simulink model "example12_3"  (R2023b)
settings: Solver=FixedStepAuto  StartTime=0.0  StopTime=1000  FixedStep=0.01  RelTol=1e-3
InitFcn:
  | example12_3_param;
values from neighbouring files (symbols this model uses):
  A = [1 1 ; 0 1]    [example12_3_param.m]
  B = [0 ; 1]    [example12_3_param.m]
  Bw = [1; 1]    [example12_3_param.m]
  C = [1 0]    [example12_3_param.m]
  G = lqe(A,Bw,C,Qw,Rw)    [example12_3_param.m]
  K = lqr(A,B,Q,R)    [example12_3_param.m]
  x0 = [0.2; 0.75]    [example12_3_param.m]
  xhat0 = [0; 0]    [example12_3_param.m]
libraries: simulink x2
settings Model: LastModifiedBy=vcichella
settings OptimizationCC: ReuseModelBlockBuffer=off
settings DebuggingCC: UnconnectedInputMsg=warning  UnconnectedOutputMsg=warning  UnconnectedLineMsg=warning
settings ModelReferenceCC: EnableRefExpFcnMdlSchedulingChecks=on
settings RTWCC: DLArmComputeVersion=19.05

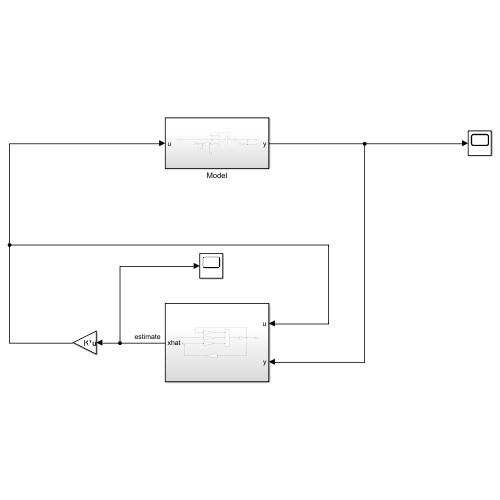
[thumbnail: Simulink's stored preview of the top-level diagram]
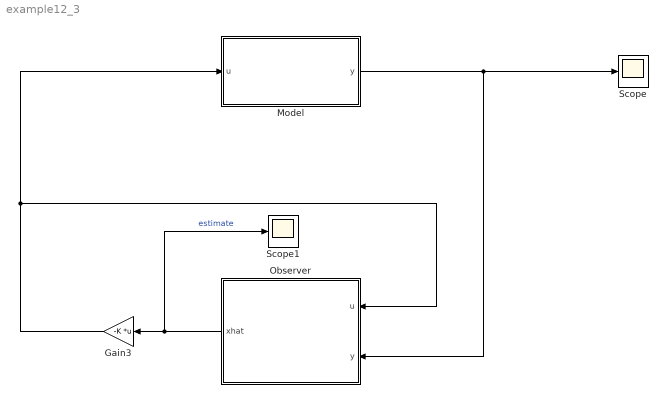
== system example12_3 ==
  Gain3 : Gain  Gain=-K  Multiplication=Matrix(K*u)
  Model : Subsystem
  Observer : Subsystem
  Scope : Scope
  Scope1 : Scope
  wires:
  Observer/1(xhat) -> Scope1/1, Gain3/1  "estimate"
  Gain3/1 -> Model/1(u), Observer/1(u)
  Model/1(y) -> Scope/1, Observer/2(y)

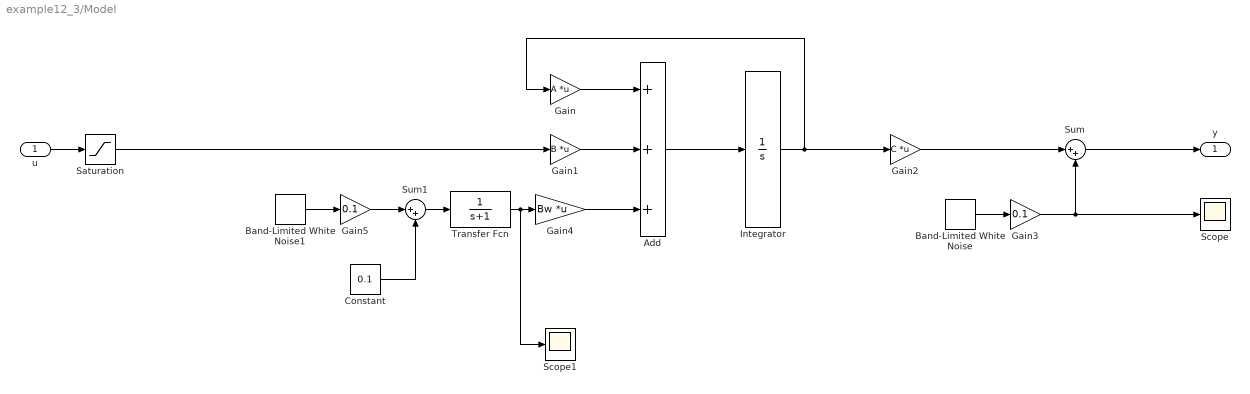
== system example12_3/Model ==
  u : Inport
  Add : Sum  Inputs=+++
  Band-Limited White Noise : simulink/Sources/Band-Limited White Noise  Cov=[0.1]  Ts=0.1  seed=[23341]
  Band-Limited White Noise1 : simulink/Sources/Band-Limited White Noise  Cov=[0.1]  Ts=0.1  seed=[23341]
  Constant : Constant  Value=0.1
  Gain : Gain  Gain=A  Multiplication=Matrix(K*u)
  Gain1 : Gain  Gain=B  Multiplication=Matrix(K*u)
  Gain2 : Gain  Gain=C  Multiplication=Matrix(K*u)
  Gain3 : Gain  Gain=0.1
  Gain4 : Gain  Gain=Bw  Multiplication=Matrix(K*u)
  Gain5 : Gain  Gain=0.1
  Integrator : Integrator  InitialCondition=x0
  Saturation : Saturate  UpperLimit=10  LowerLimit=-10
  Scope : Scope
  Scope1 : Scope
  Sum : Sum  Inputs=|++
  Sum1 : Sum  Inputs=|++
  Transfer Fcn : TransferFcn  Denominator=[1 1]
  y : Outport
  wires:
  Gain1/1 -> Add/2
  Add/1 -> Integrator/1
  Integrator/1 -> Gain2/1, Gain/1
  u/1 -> Saturation/1
  Gain/1 -> Add/1
  Gain2/1 -> Sum/1
  Sum/1 -> y/1
  Band-Limited White Noise/1 -> Gain3/1
  Gain3/1 -> Scope/1, Sum/2
  Gain4/1 -> Add/3
  Band-Limited White Noise1/1 -> Gain5/1
  Gain5/1 -> Sum1/1
  Constant/1 -> Sum1/2
  Sum1/1 -> Transfer Fcn/1
  Transfer Fcn/1 -> Scope1/1, Gain4/1
  Saturation/1 -> Gain1/1

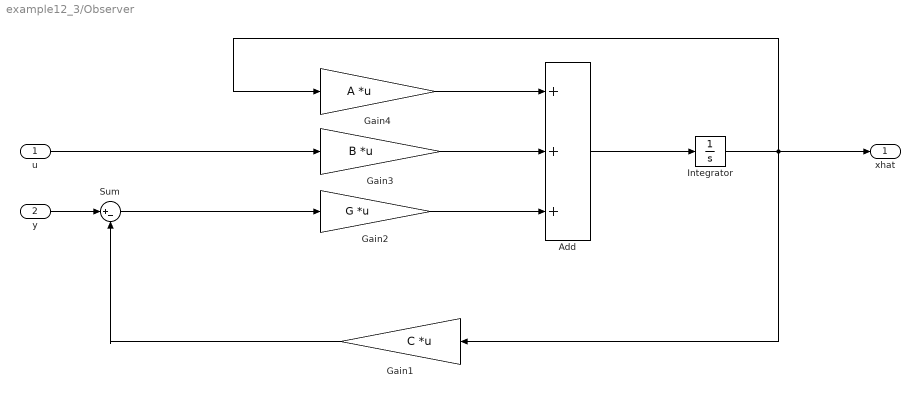
== system example12_3/Observer ==
  u : Inport
  y : Inport  Port=2
  Add : Sum  Inputs=+++
  Gain1 : Gain  Gain=C  Multiplication=Matrix(K*u)
  Gain2 : Gain  Gain=G  Multiplication=Matrix(K*u)
  Gain3 : Gain  Gain=B  Multiplication=Matrix(K*u)
  Gain4 : Gain  Gain=A  Multiplication=Matrix(K*u)
  Integrator : Integrator  InitialCondition=xhat0
  Sum : Sum  Inputs=|+-
  xhat : Outport
  wires:
  Gain3/1 -> Add/2
  u/1 -> Gain3/1
  Gain2/1 -> Add/3
  Gain4/1 -> Add/1
  Add/1 -> Integrator/1
  y/1 -> Sum/1
  Sum/1 -> Gain2/1
  Integrator/1 -> xhat/1, Gain1/1, Gain4/1
  Gain1/1 -> Sum/2
